simulink model "sensors"  (R2026a)
settings: configuration reference "standardSILConfiguraitonParams" (kept outside this file)
values from neighbouring files (symbols this model uses):
  INS_VARIANT = 1    [setUpSensors.m]
settings Model: Creator=GTAR  LastModifiedBy=Usuario
settings ConfigSetRef: SourceName=standardSILConfiguraitonParams  SourceLocation=Base Workspace

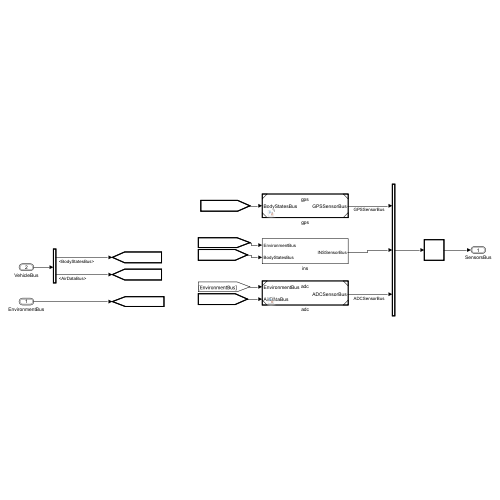
[thumbnail: Simulink's stored preview of the top-level diagram]
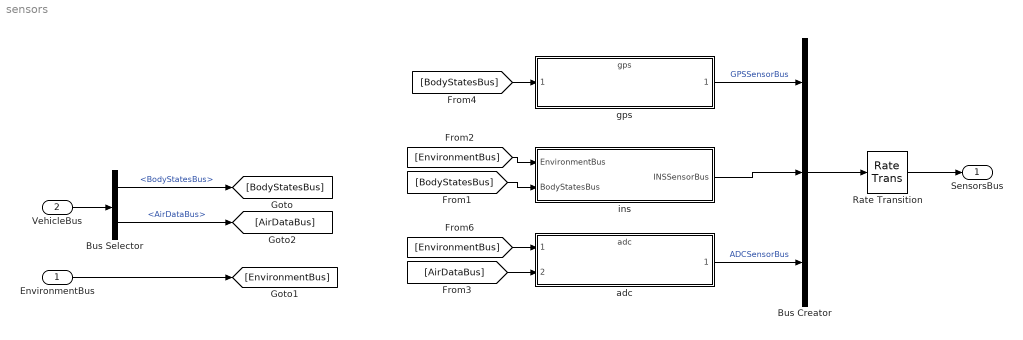
== system sensors ==
  EnvironmentBus : Inport  OutDataTypeStr=Bus: EnvironmentBus
  VehicleBus : Inport  Port=2  OutDataTypeStr=Bus: VehicleBus
  Bus Creator : BusCreator  Inputs=3  OutDataTypeStr=Bus: SensorsBus
      settings: InheritFromInputs=off
  Bus Selector : BusSelector  OutputSignals=BodyStatesBus,AirDataBus
  Rate Transition : RateTransition
  adc : ModelReference  ModelNameDialog=adc.slx  SimulationMode=Normal  ModelReferenceVersion=1.68
  gps : ModelReference  ModelNameDialog=gps.slx  SimulationMode=Normal  ModelReferenceVersion=1.43
  ins : Subsystem
  SensorsBus : Outport  OutDataTypeStr=Bus: SensorsBus  BusOutputAsStruct=on
  wires:
  Bus Creator/1 -> Rate Transition/1
  VehicleBus/1 -> Bus Selector/1
  Bus Selector/1 -> [BodyStatesBus]  "<BodyStatesBus>"
  EnvironmentBus/1 -> [EnvironmentBus]
  [AirDataBus] -> adc/2
  [EnvironmentBus] -> adc/1
  [BodyStatesBus] -> gps/1
  Bus Selector/2 -> [AirDataBus]  "<AirDataBus>"
  Rate Transition/1 -> SensorsBus/1
  gps/1 -> Bus Creator/1  "GPSSensorBus"
  adc/1 -> Bus Creator/3  "ADCSensorBus"
  [EnvironmentBus] -> ins/1(EnvironmentBus)
  [BodyStatesBus] -> ins/2(BodyStatesBus)
  ins/1(INSSensorBus) -> Bus Creator/2

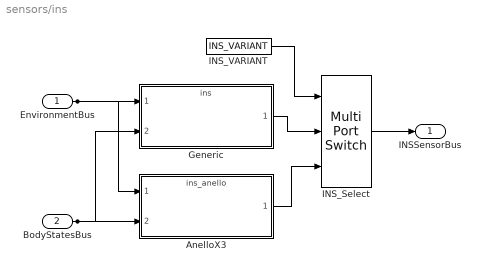
== system sensors/ins ==
  EnvironmentBus : Inport
  BodyStatesBus : Inport  Port=2
  AnelloX3 : ModelReference  ModelNameDialog=ins_anello.slx  SimulationMode=Normal  ModelReferenceVersion=1.1
  Generic : ModelReference  ModelNameDialog=ins.slx  SimulationMode=Normal  ModelReferenceVersion=1.45
  INS_Select : MultiPortSwitch  Inputs=2  SaturateOnIntegerOverflow=off  InputSameDT=off
  INS_VARIANT : Constant  Value=INS_VARIANT
  INSSensorBus : Outport
  wires:
  EnvironmentBus/1 -> Generic/1, AnelloX3/1
  BodyStatesBus/1 -> Generic/2, AnelloX3/2
  INS_VARIANT/1 -> INS_Select/1
  INS_Select/1 -> INSSensorBus/1
  AnelloX3/1 -> INS_Select/3
  Generic/1 -> INS_Select/2
